simulink model "schema_robot_2"  (R2018b)
settings: Solver=VariableStepAuto  StartTime=0.0  StopTime=10.0  RelTol=1e-3  EnableMultiTasking=on
values from neighbouring files (symbols this model uses):
  RB = struct()    [robot_numeric.m]    (also in robot_numeric_2.m)
libraries: cstblocks x2
settings Model: Creator=ygorra  LastModifiedBy=msalimi
settings OptimizationCC: LifeSpan=inf
settings DebuggingCC: SFUnexpectedBacktrackingDiag=warning  SFNoUnconditionalDefaultTransitionDiag=warning  SFExecutionAtInitializationDiag=none
settings SFSimCC: SimUseLocalCustomCode=off
settings RTWCC: RTWUseLocalCustomCode=off
settings CodeAppCC: StateflowObjectComments=on
settings GRTTargetCC: TargetLangStandard=C89/C90 (ANSI)  GeneratePreprocessorConditionals=Disable all
settings ConfigComp: CovMetricSettings=dw  CovHtmlReporting=on  CovSaveCumulativeToWorkspaceVar=on  CovSaveSingleToWorkspaceVar=on  CovExternalEMLEnable=off

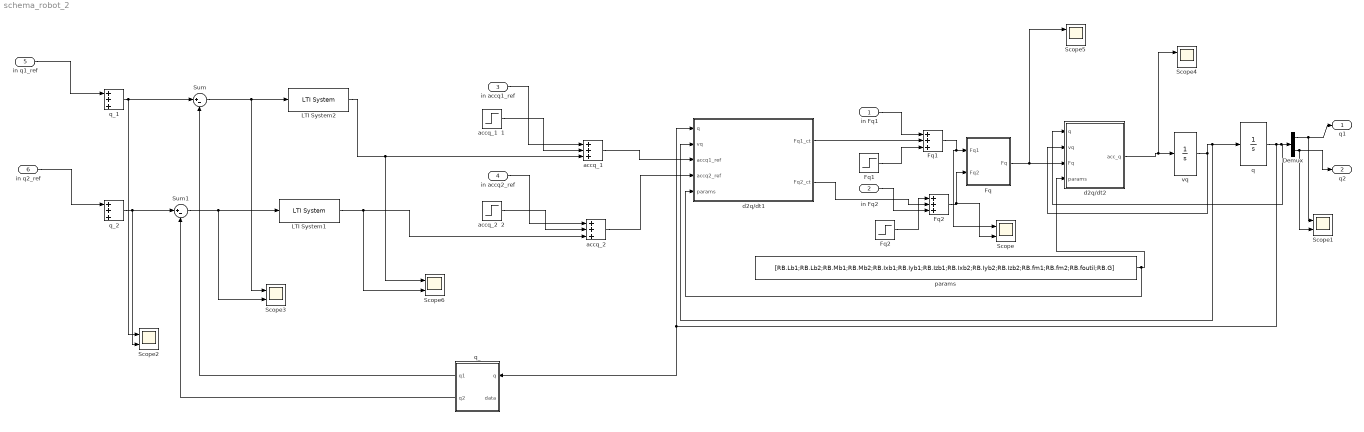
== system schema_robot_2 ==
  in Fq1 : Inport
  in Fq2 : Inport  Port=2
  in accq1_ref : Inport  Port=3
  in accq2_ref : Inport  Port=4
  in q1_ref : Inport  Port=5
  in q2_ref : Inport  Port=6
  Demux : Demux  Outputs=2
  Fq : MATLAB Function  TreatAsAtomicUnit=on
  "Fq1  " : Step  Time=RB.t_Fq1  Before=RB.Fq1_0  After=RB.Fq1_1  SampleTime=0
  "Fq1   " : Sum  Inputs=+++
  "Fq2 " : Step  Time=RB.t_Fq2  Before=RB.Fq2_0  After=RB.Fq2_1  SampleTime=0
  "Fq2   " : Sum  Inputs=+++
  LTI System1 : cstblocks/LTI System  sys=K  IC=[]
  LTI System2 : cstblocks/LTI System  sys=K  IC=[]
  Scope{,1..6} (7 alike) : Scope  NumInputPorts=2
  Sum : Sum  Inputs=|+-
  Sum1 : Sum  Inputs=|+-
  accq_1 : Sum  Inputs=+++
  accq_1  1 : Step  Time=RB.t_Fq1  SampleTime=0
  accq_2 : Sum  Inputs=+++
  accq_2  2 : Step  Time=RB.t_Fq1  SampleTime=0
  d2q/dt1 : MATLAB Function  TreatAsAtomicUnit=on
  d2q/dt2 : MATLAB Function  TreatAsAtomicUnit=on
  params : Constant  Value=[RB.Lb1;RB.Lb2;RB.Mb1;RB.Mb2;RB.Ixb1;RB.Iyb1;RB.Izb1;RB.Ixb2;RB.Iyb2;RB.Izb2;RB.fm1;RB.fm2;RB.foutil;RB.G]
  q : Integrator  InitialCondition=[RB.q1_init;RB.q2_init]  ContinuousStateAttributes='q'
  q_ : MATLAB Function  TreatAsAtomicUnit=on
  q_1 : Sum  Inputs=+++
  q_2 : Sum  Inputs=+++
  vq : Integrator  InitialCondition=[RB.vq1_init;RB.vq2_init]  ContinuousStateAttributes='vq'
  q1 : Outport
  q2 : Outport  Port=2
  wires:
  Demux/1 -> Scope1/1, q1/1
  d2q/dt2/1(acc_q) -> Scope4/1, vq/1
  vq/1 -> d2q/dt2/2(vq), d2q/dt1/2(vq), q/1
  q/1 -> d2q/dt1/1(q), q_/1(q), Demux/1, d2q/dt2/1(q)
  Fq/1(Fq) -> Scope5/1, d2q/dt2/3(Fq)
  params/1 -> d2q/dt1/5(params), d2q/dt2/4(params)
  "Fq1   "/1 -> Fq/1(Fq1), Scope/1
  "Fq2   "/1 -> Scope/2, Fq/2(Fq2)
  Demux/2 -> Scope1/2, q2/1
  d2q/dt1/1(Fq1_ct) -> "Fq1   "/2
  d2q/dt1/2(Fq2_ct) -> "Fq2   "/2
  accq_1/1 -> d2q/dt1/3(accq1_ref)
  accq_2/1 -> d2q/dt1/4(accq2_ref)
  Sum/1 -> LTI System2/1, Scope3/1
  Sum1/1 -> LTI System1/1, Scope3/2
  q_/1(q1) -> Sum/2
  q_/2(q2) -> Sum1/2
  q_1/1 -> Sum/1, Scope2/1
  q_2/1 -> Scope2/2, Sum1/1
  LTI System2/1 -> Scope6/1, accq_1/3
  LTI System1/1 -> Scope6/2, accq_2/3
  in q1_ref/1 -> q_1/1
  in q2_ref/1 -> q_2/1
  accq_2  2/1 -> accq_2/2
  in accq2_ref/1 -> accq_2/1
  accq_1  1/1 -> accq_1/2
  in accq1_ref/1 -> accq_1/1
  in Fq2/1 -> "Fq2   "/3
  "Fq1  "/1 -> "Fq1   "/3
  in Fq1/1 -> "Fq1   "/1
  "Fq2 "/1 -> "Fq2   "/1

== matlab function schema_robot_2/Fq ==
  data: Fq1 input; Fq2 input; Fq output
function Fq=Fq_(Fq1,Fq2)
    Fq=[Fq1;Fq2];
end

== matlab function schema_robot_2/d2q//dt2 ==
  data: q input; vq input; Fq input; acc_q output; params input
function acc_q=clc_accq(q,vq,Fq,params)
    q1=q(1);    
    q2=q(2);
    vq1=vq(1);
    vq2=vq(2);
    Lb1=params(1);
    Lb2=params(2);
    Mb1=params(3);
    Mb2=params(4);
    Ixb1=params(5);
    Iyb1=params(6);
    Izb1=params(7);
    Ixb2=params(8);
    Iyb2=params(9);
    Izb2=params(10);
    fm1=params(11);
    fm2=params(12);
    foutil=params(13);
    G=params(14);
    A= clc_A(q1,q2,Lb1,Lb2,Mb1,Mb2,Ixb1,Iyb1,Izb1,Ixb2,Iyb2,Izb2,fm1,fm2,foutil,G);
    H= clc_H(q1,q2,vq1,vq2,Lb1,Lb2,Mb1,Mb2,Ixb1,Iyb1,Izb1,Ixb2,Iyb2,Izb2,fm1,fm2,foutil,G);
    acc_q=pinv(A)*(Fq-H);
end

== matlab function schema_robot_2/d2q//dt1 ==
  data: q input; vq input; accq1_ref input; accq2_ref input; Fq1_ct output; params input; Fq2_ct output
function [Fq1_ct, Fq2_ct]=clc_accq(q,vq,accq1_ref, accq2_ref,params)
    q1=q(1);    
    q2=q(2);
    vq1=vq(1);
    vq2=vq(2);
    Lb1=params(1);
    Lb2=params(2);
    Mb1=params(3);
    Mb2=params(4);
    Ixb1=params(5);
    Iyb1=params(6);
    Izb1=params(7);
    Ixb2=params(8);
    Iyb2=params(9);
    Izb2=params(10);
    fm1=params(11);
    fm2=params(12);
    foutil=params(13);
    G=params(14);
    A= clc_A(q1,q2,Lb1,Lb2,Mb1,Mb2,Ixb1,Iyb1,Izb1,Ixb2,Iyb2,Izb2,fm1,fm2,foutil,G);
    H= clc_H(q1,q2,vq1,vq2,Lb1,Lb2,Mb1,Mb2,Ixb1,Iyb1,Izb1,Ixb2,Iyb2,Izb2,fm1,fm2,foutil,G);
    
    accq = [accq1_ref; accq2_ref];
    
    Fq = A * accq + H;
    Fq1_ct = Fq(1,1);
    Fq2_ct = Fq(2,1);
end

== matlab function schema_robot_2/q_ ==
  data: q input; q1 output; q2 output; data input
function [q1, q2]=q_(q, data)
    q1 = q(1);
    q2 = q(2);
end
